simulink model "Velocity_Simple_Model"  (R2018b)
settings: Solver=VariableStepAuto  StartTime=0.0  StopTime=120  RelTol=1e-3
undefined symbols (not defined in the file): b, m
settings Model: Creator=Kacpix  LastModifiedBy=Kacpix

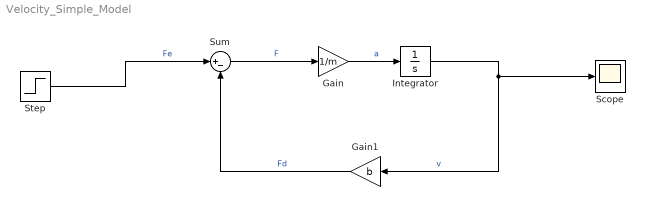
== system Velocity_Simple_Model ==
  Gain : Gain  Gain=1/m
  Gain1 : Gain  Gain=b
  Integrator : Integrator
  Scope : Scope
  Step : Step  After=u  SampleTime=0
  Sum : Sum  Inputs=|+-
  wires:
  Integrator/1 -> Scope/1, Gain1/1  "v"
  Gain/1 -> Integrator/1  "a"
  Sum/1 -> Gain/1  "F"
  Step/1 -> Sum/1  "Fe"
  Gain1/1 -> Sum/2  "Fd"
